simulink model "SG__MDL_IO397"  (R2020a)
settings: Solver=FixedStepAuto  StartTime=0.0  StopTime=Inf  RelTol=1e-3  EnableMultiTasking=on
undefined symbols (not defined in the file): ff, tmax
libraries: dspfdesign x4, slrtlib x2, SG_library x1, simulink x1, dspsrcs4 x1
settings Model: SimulationMode=external  Creator=padlewsk  LastModifiedBy=padlewsk
settings SolverCC: ConcurrentTasks=on  AutoInsertRateTranBlk=on
settings DataIOCC: SaveFormat=StructureWithTime
settings OptimizationCC: BlockReduction=off  OptimizeBlockIOStorage=off
settings DebuggingCC: SFMachineParentedDataDiag=error
settings HardwareCC: ProdBitPerPointer=32  ProdBitPerSizeT=32  ProdBitPerPtrDiffT=32  ProdLargestAtomicFloat=None  ProdWordSize=32  ProdLongLongMode=on  ProdHWDeviceType=Generic->32-bit x86 compatible
settings RTWCC: Description=Simulink Real-Time  SystemTargetFile=slrt.tlc  TemplateMakefile=slrt_default_tmf  RTWVerbose=off  CodeExecutionProfiling=on  RTWCompilerOptimization=on
settings SimulinkRealTimeCC: SupportVariableSizeSignals=on  RL32LogTETModifier=off  xPCConcurrentTasks=on

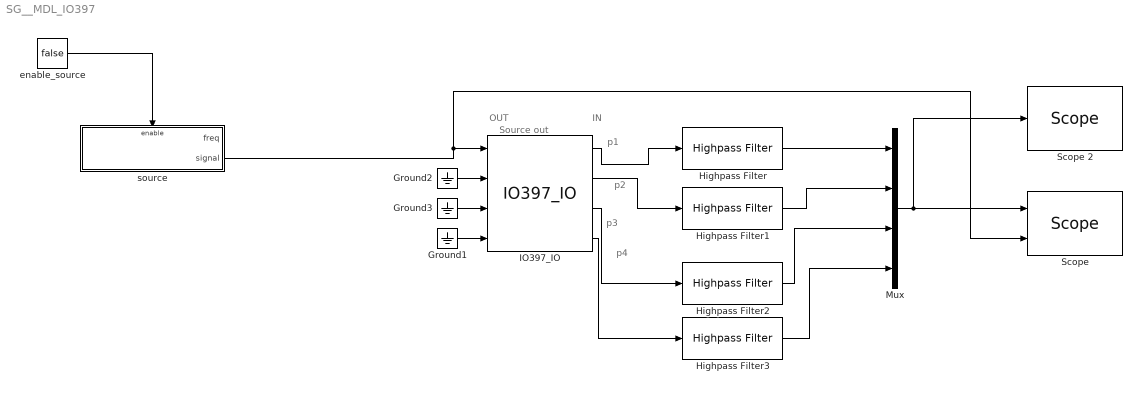
== system SG__MDL_IO397 ==
  note: p2
  note: p3
  note: p1
  note: Source out
  note: IN
  note: OUT
  note: p4
  Ground1 : Ground
  Ground2 : Ground
  Ground3 : Ground
  Highpass Filter : dspfdesign/Highpass Filter  FilterType=IIR  DesignForMinimumOrder=off  FilterOrder=4  StopbandFrequency=8e3  PassbandFrequency=5  StopbandAttenuation=80  PassbandRipple=0.1  InheritSampleRate=off  SampleRate=30000  SimulateUsing=Interpreted execution  roundingMode=Floor  coeffsDataTypeStr=fixdt(1,16)
  Highpass Filter1 : dspfdesign/Highpass Filter  FilterType=IIR  DesignForMinimumOrder=off  FilterOrder=4  StopbandFrequency=8e3  PassbandFrequency=5  StopbandAttenuation=80  PassbandRipple=0.1  InheritSampleRate=off  SampleRate=30000  SimulateUsing=Interpreted execution  roundingMode=Floor  coeffsDataTypeStr=fixdt(1,16)
  Highpass Filter2 : dspfdesign/Highpass Filter  FilterType=IIR  DesignForMinimumOrder=off  FilterOrder=4  StopbandFrequency=8e3  PassbandFrequency=5  StopbandAttenuation=80  PassbandRipple=0.1  InheritSampleRate=off  SampleRate=30000  SimulateUsing=Interpreted execution  roundingMode=Floor  coeffsDataTypeStr=fixdt(1,16)
  Highpass Filter3 : dspfdesign/Highpass Filter  FilterType=IIR  DesignForMinimumOrder=on  FilterOrder=50  StopbandFrequency=4  PassbandFrequency=5  StopbandAttenuation=80  PassbandRipple=0.1  InheritSampleRate=off  SampleRate=30000  SimulateUsing=Interpreted execution  roundingMode=Floor  coeffsDataTypeStr=fixdt(1,16)
  IO397_IO : SG_library/Built elements/IO397_IO
      settings: SourceProductName=Custom Speedgoat implementations
  Mux : Mux
  "Scope " : slrtlib/Displays and Logging/Scope   scopeno=2  scopetype=Host  autostart=on  viewmode=Graphical redraw  formatstr='%15.6f'  grid=on  ylimits=[0,0]  nosamples=800000  noprepostsamples=0  interleave=1  triggermode=Signal triggering  triggersignal=1  trigsignalfromport=on  triggerlevel=0.001  triggerslope=Either  triggerscope=1  triggersample=0  filename=data.dat  mode=Lazy  writesize=512  autorestart=off  dynamicfilemode=off  maxwritefilesize=512*1024^2
  Scope 2 : slrtlib/Displays and Logging/Scope   scopeno=1  scopetype=Target  autostart=on  viewmode=Graphical redraw  formatstr='%15.6f'  grid=on  ylimits=[-10,10]  nosamples=800000  noprepostsamples=0  interleave=1  triggermode=FreeRun  triggersignal=1  trigsignalfromport=off  triggerlevel=0.45  triggerslope=Either  triggerscope=1  triggersample=0  filename=data.dat  mode=Lazy  writesize=512  autorestart=off  dynamicfilemode=off  maxwritefilesize=512*1024^2
  enable_source : Constant  Value=false  SampleTime=-1
  source : Subsystem  TreatAsAtomicUnit=on
  wires:
  enable_source/1 -> source/Enable
  Mux/1 -> Scope 2/1, "Scope "/1
  Highpass Filter2/1 -> Mux/3
  source/2(signal) -> "Scope "/2, IO397_IO/1
  Highpass Filter3/1 -> Mux/4
  IO397_IO/1 -> Highpass Filter/1
  IO397_IO/2 -> Highpass Filter1/1
  IO397_IO/3 -> Highpass Filter2/1
  IO397_IO/4 -> Highpass Filter3/1
  Ground2/1 -> IO397_IO/2
  Highpass Filter/1 -> Mux/1
  Highpass Filter1/1 -> Mux/2
  Ground1/1 -> IO397_IO/4
  Ground3/1 -> IO397_IO/3

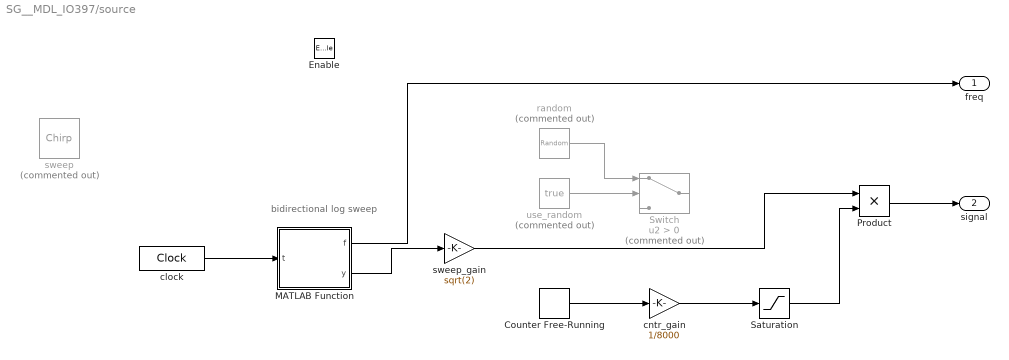
== system SG__MDL_IO397/source ==
  note: bidirectional log sweep
  Enable : EnablePort  StatesWhenEnabling=reset
  Counter Free-Running : simulink/Sources/Counter Free-Running  NumBits=32  tsamp=-1
  MATLAB Function : MATLAB Function  TreatAsAtomicUnit=on
  Product : Product
  Saturation : Saturate  UpperLimit=1  LowerLimit=0
  Switch : Switch  Commented=on  Criteria=u2 > Threshold
  clock : DigitalClock  SampleTime=0.01
  cntr_gain : Gain  Gain=1/8000  ParamDataTypeStr=double
  random : RandomNumber  Commented=on  Variance=0.5  SampleTime=3.3333e-05
  sweep : dspsrcs4/Chirp  Commented=on  sweep=Logarithmic  mode=Bidirectional  f0=50  f1=500  t1=2  Tsweep=2  phase=0  Ts=3.3333e-05  spf=1  datatype=Double  OutputFrames=off
  sweep_gain : Gain  Gain=sqrt(2)
  use_random : Constant  Commented=on  Value=true  SampleTime=-1
  freq : Outport
  signal : Outport  Port=2  OutputWhenDisabled=reset  InitialOutput=0  VectorParamsAs1DForOutWhenUnconnected=off
  wires:
  Saturation/1 -> Product/2
  cntr_gain/1 -> Saturation/1
  use_random/1 -> Switch/2
  Counter Free-Running/1 -> cntr_gain/1
  Product/1 -> signal/1
  random/1 -> Switch/1
  MATLAB Function/2(y) -> sweep_gain/1
  clock/1 -> MATLAB Function/1(t)
  MATLAB Function/1(f) -> freq/1
  sweep_gain/1 -> Product/1

== matlab function SG__MDL_IO397/source/MATLAB Function ==
  data: f output; t input; y output; tmax parameter; fi parameter; ff parameter
function [f,y] = fcn(t,tmax, fi, ff)

x = t/tmax;

if mod(floor(x), 2) == 0
    % up
    dir = 1;
    x = mod(x, 1);
else
    % down
    dir = -1;
    x = 1 - mod(x, 1);
end

%f = fi + ((ff-fi)/tmax).*t(1:N/2); %%%linear frequency vector
%f = fi + ((ff-fi)/tmax).*t(1:N/2).^2; %%%quadratic frequency vector
%f = fi + 10.^(log10(ff-fi)/(tmax/2).*t(1:N/2)); %%%logarithmic frequency vector
f = fi + 10.^(log10(ff-fi)*x); %%%logarithmic frequency vector
y = sin(2*pi*f*x*tmax);
